simulink model "QET_KV"  (R2015b)
settings: Solver=ode4  SolverMode=SingleTasking  StartTime=0.0  StopTime=inf  FixedStep=Ts  RelTol=1e-3
values from neighbouring files (symbols this model uses):
  F_M_Direction = [1 1 1 -1 -1 -1]    [Config_StepperMotor.m]
  NanoCal7342 = [-0.945276141167 14.673559188843 0.251662999392 -14.892200469971 -0.854624807835 0.034513175488 ... (first row only)    [NanoCalibration.m]
  Resolution = (360/200 * 1/64)    (= 0.028125)    [Config_StepperMotor.m]
undefined symbols (not defined in the file or in its folder): AnalogPos_to_deg, anVE, anVE_GBC_Kbi, anVE_GBC_Kbp, anVE_K_int, anVE_Position_Gain_inv, anVE_Saturation, B, Chirp_Amplitude, Chirp_Freq_Max, Chirp_Freq_Min, Chirp_Period, Chirp_Time_Start, Chirp_Type, delay, Delta, DO_DG409_A0, DO_DG409_A1, Driver_Type, HIL, K, K_gyro, Kd, Kp, lambda, mag, Pos_Final, Pos_Init, Pos_Threshold, PSoC_Freq, qc_get_step_size, Stabilization_Period, Test_type, Times, Torque_Threshold, Ts, Ts_loop, VE_Platform, VE_Type
libraries: quarc_library x22, simulink x13, dspsigops x1
(part 2 of 3)

== system QET_KV/Stability Check and Control ==
  Clock : Clock
  Display : Display
  Display1 : Display
  Initial and Final Condition Control : Subsystem
  Stability Check : Subsystem
  To Workspace2 : ToWorkspace  VariableName=is_stable_vec  SampleTime=-1
      settings: Save2DSignal=2-D array (concatenate along first dimension)
  Switch-State : Outport
  Stable Torque : Outport  Port=2
  tag scope: StabCheck_Pos=global, StabCheck_State=global, is_stable_vec=global
  wires:
  Initial and Final Condition Control/2(Stable Torque) -> Stable Torque/1  "PD"
  Clock/1 -> Display/1, Initial and Final Condition Control/1(Clock), Stability Check/2(Clock)
  Stability Check/1(is_stable) -> [is_stable_vec], To Workspace2/1, Initial and Final Condition Control/2(is_stable), Display1/1
  Initial and Final Condition Control/1(Switch-State) -> [StabCheck_State], Switch-State/1
  Initial and Final Condition Control/4(Pos_Final) -> Stability Check/1(Pos_Final)
  Initial and Final Condition Control/3(Pos_PD) -> [StabCheck_Pos]

== system QET_KV/Step with Rate Limiter ==
  In1 : Inport
  Add1 : Sum  Inputs=+-
  Constant7 : Constant  Value=0
  Manual Switch2 : ManualSwitch
  Multiport Switch2 : MultiPortSwitch  Inputs=2  DataPortForDefault=Additional data port  SampleTime=Ts
  Pulse : Scope
  Rate Limiter : RateLimiter  RisingSlewLimit=100 * pi/180  FallingSlewLimit=-100 * pi/180  SampleTimeMode=inherited
  Scope1 : Scope
  Scope2 : Scope
  Out1 : Outport
  wires:
  In1/1 -> Add1/1, Multiport Switch2/2
  Multiport Switch2/1 -> Scope2/1, Manual Switch2/2, Rate Limiter/1
  Add1/1 -> Pulse/1, Out1/1
  Constant7/1 -> Multiport Switch2/4, Multiport Switch2/3
  [StabCheck_State] -> Scope1/1, Multiport Switch2/1
  Rate Limiter/1 -> Manual Switch2/1
  Manual Switch2/1 -> Add1/2

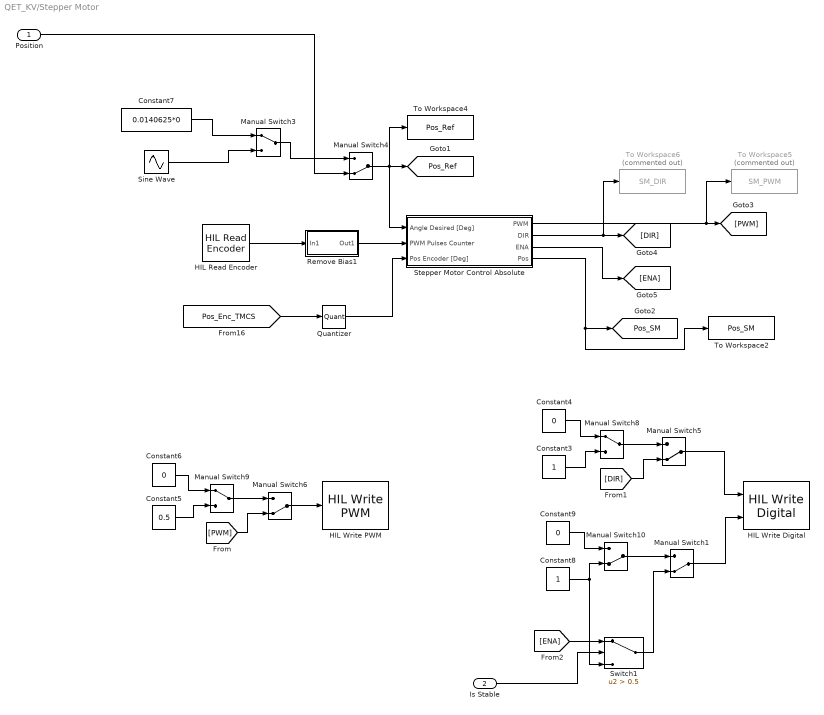
== system QET_KV/Stepper Motor ==
  Position : Inport
  Is Stable : Inport  Port=2
  Constant3 : Constant
  Constant4 : Constant  Value=0
  Constant5 : Constant  Value=0.5
  Constant6 : Constant  Value=0
  Constant7 : Constant  Value=0.0140625*0
  Constant8 : Constant
  Constant9 : Constant  Value=0
  HIL Read Encoder : quarc_library/Data Acquisition/Generic/Immediate I//O/HIL Read Encoder  object_name=HIL-1  channels=[0]  sample_time=qc_get_step_size  active=on  vector_output=off  data_type_mode=Inherit via back propagation  data_type=double
  HIL Write Digital : quarc_library/Data Acquisition/Generic/Immediate I//O/HIL Write Digital  object_name=HIL-1  channels=[0 7]  sample_time=-1  active=off  vector_input=off
  HIL Write PWM : quarc_library/Data Acquisition/Generic/Immediate I//O/HIL Write PWM  object_name=HIL-1  channels=[1]  sample_time=Ts  active=off  vector_input=off
      settings: AttributesFormatString=(%<object_name>)
  Manual Switch{1,4..6,10} (5 alike) : ManualSwitch  CurrentSetting=0
  Manual Switch3 : ManualSwitch
  Manual Switch8 : ManualSwitch
  Manual Switch9 : ManualSwitch
  Quantizer : Quantizer  QuantizationInterval=Resolution  SampleTime=Ts
  Remove Bias1 : Subsystem
  Sine Wave : Sin  Amplitude=0.0140625*5  Frequency=2*pi*1  SampleTime=0
  Stepper Motor Control Absolute : Subsystem
  Switch1 : Switch  Criteria=u2 > Threshold  Threshold=0.5
  To Workspace2 : ToWorkspace  VariableName=Pos_SM  SampleTime=-1
      settings: Save2DSignal=2-D array (concatenate along first dimension)
  To Workspace4 : ToWorkspace  VariableName=Pos_Ref  SampleTime=-1
      settings: Save2DSignal=2-D array (concatenate along first dimension)
  To Workspace5 : ToWorkspace  Commented=on  VariableName=SM_PWM  SampleTime=-1
      settings: Save2DSignal=2-D array (concatenate along first dimension)
  To Workspace6 : ToWorkspace  Commented=on  VariableName=SM_DIR  SampleTime=-1
      settings: Save2DSignal=2-D array (concatenate along first dimension)
  tag scope: Pos_Ref=global, Pos_SM=global
  wires:
  Manual Switch9/1 -> Manual Switch6/1
  Manual Switch3/1 -> Manual Switch4/1
  Manual Switch8/1 -> Manual Switch5/1
  Manual Switch5/1 -> HIL Write Digital/1
  Manual Switch6/1 -> HIL Write PWM/1
  Sine Wave/1 -> Manual Switch3/2
  [PWM] -> Manual Switch6/2
  [DIR] -> Manual Switch5/2
  Manual Switch4/1 -> [Pos_Ref], Stepper Motor Control Absolute/1(Angle Desired [Deg]), To Workspace4/1
  Stepper Motor Control Absolute/1(PWM) -> [PWM], To Workspace5/1
  Stepper Motor Control Absolute/2(DIR) -> [DIR], To Workspace6/1
  HIL Read Encoder/1 -> Remove Bias1/1(In1)
  Stepper Motor Control Absolute/4(Pos) -> To Workspace2/1, [Pos_SM]
  Position/1 -> Manual Switch4/2
  Constant7/1 -> Manual Switch3/1
  Remove Bias1/1(Out1) -> Stepper Motor Control Absolute/2(PWM Pulses Counter)
  [Pos_Enc_TMCS] -> Quantizer/1
  Quantizer/1 -> Stepper Motor Control Absolute/3(Pos Encoder [Deg])
  Constant3/1 -> Manual Switch8/2
  Constant4/1 -> Manual Switch8/1
  Constant6/1 -> Manual Switch9/1
  Constant5/1 -> Manual Switch9/2
  Constant9/1 -> Manual Switch10/1
  Manual Switch10/1 -> Manual Switch1/1
  Manual Switch1/1 -> HIL Write Digital/2
  Stepper Motor Control Absolute/3(ENA) -> [ENA]
  Constant8/1 -> Switch1/3, Manual Switch10/2
  [ENA] -> Switch1/1
  Is Stable/1 -> Switch1/2
  Switch1/1 -> Manual Switch1/2

== system QET_KV/Time Enable1 ==
  In1 : Inport
  Product2 : Product  Inputs=3
  Step4 : Step  Time=Chirp_Time_Start-0.007  SampleTime=Ts
  Step5 : Step  Time=Chirp_Period+1.5  Before=1  After=0  SampleTime=Ts
  Out1 : Outport
  wires:
  Step5/1 -> Product2/3
  Product2/1 -> Out1/1
  In1/1 -> Product2/1
  Step4/1 -> Product2/2

== system QET_KV/Torques ==
  Display : Display
  Gain : Gain  Gain=-1
  Mux1 : Mux  Inputs=2
  Mux2 : Mux  Inputs=2
  Mux6 : Mux
  Torque F/T Sensor : Scope
  Torques : Scope
  Voltage Applied : Scope
  wires:
  Mux6/1 -> Display/1, Torques/1
  [Torque_Haptic] -> Mux6/1  "VE"
  [Torque_Current_QET2] -> Mux6/2  "Current QET2"
  [Torque_Current_AMC] -> Mux6/3  "Current AMC"
  [Torque_Current_CD1] -> Mux6/4  "Current CD1"
  Mux1/1 -> Torque F/T Sensor/1
  [Torque_Current_CD1] -> Mux1/2
  [Torque_Nano25] -> Gain/1
  Gain/1 -> Mux1/1
  [anVE_Output_Voltage] -> Mux2/1
  [DC_Motor_Analog] -> Mux2/2
  Mux2/1 -> Voltage Applied/1

== system QET_KV/Virtual Environment ==
  Position : Inport
  Constant10 : Constant
  Constant5 : Constant  Value=delay
  Constant9 : Constant  Value=VE_Type
  Deg to Rad : Gain  Gain=pi/180
  Force VE Delay : Scope
  Manual Switch2 : ManualSwitch
  Manual Switch4 : ManualSwitch
  Multiport Switch2 : MultiPortSwitch  DataPortForDefault=Additional data port  SampleTime=Ts
  Mux7 : Mux  Inputs=2
  To Workspace1 : ToWorkspace  VariableName=Torque_VE_Both  SampleTime=-1
      settings: Save2DSignal=2-D array (concatenate along first dimension)
  To Workspace3 : ToWorkspace  VariableName=Torque_VE  SaveFormat=Structure With Time  SampleTime=-1
  VE_KV_BD : Subsystem
  VE_KV_GM2 : Subsystem
  VE_PV : Subsystem
  Variable Integer Delay : Delay  DelayLengthSource=Input port  DelayLengthUpperLimit=20
      settings: InputPortMap=u0,p1
  Torque : Outport
  tag scope: Torque_VE=global
  wires:
  VE_KV_BD/1(Torque) -> Multiport Switch2/2
  VE_KV_GM2/1(Torque) -> Multiport Switch2/5, Multiport Switch2/3
  Position/1 -> VE_PV/1(Position), VE_KV_GM2/1(Position), VE_KV_BD/1(Position)
  Multiport Switch2/1 -> Variable Integer Delay/1, Mux7/1, Manual Switch2/2
  Variable Integer Delay/1 -> Mux7/2, Manual Switch2/1
  Manual Switch2/1 -> Torque/1, [Torque_VE], To Workspace3/1
  Constant5/1 -> Variable Integer Delay/2
  Mux7/1 -> To Workspace1/1, Force VE Delay/1
  VE_PV/1(Torque) -> Multiport Switch2/4
  Constant9/1 -> Manual Switch4/1
  Constant10/1 -> Manual Switch4/2
  Manual Switch4/1 -> Multiport Switch2/1
  [Velocity_Gyro] -> Deg to Rad/1
  Deg to Rad/1 -> VE_PV/2(Velocity)

== system QET_KV/Analog Inputs (Analog VE)/Remove Bias w LPF ==
  In1 : Inport
  Step : Step  Time=.15  Before=1  After=0  SampleTime=qc_get_step_size
  Sum1 : Sum  Inputs=|+-
  Switch : Switch  Criteria=u2 > Threshold  Threshold=0.5  SampleTime=qc_get_step_size
  Transfer Fcn : TransferFcn  Denominator=[1/(2*pi*50) 1]
  Unit Delay : UnitDelay  SampleTime=-1
  Out1 : Outport
  wires:
  In1/1 -> Switch/1, Sum1/1
  Step/1 -> Switch/2
  Unit Delay/1 -> Switch/3
  Sum1/1 -> Out1/1
  Switch/1 -> Transfer Fcn/1, Sum1/2
  Transfer Fcn/1 -> Unit Delay/1

== system QET_KV/Analog Inputs (Analog VE)/Remove Bias2 ==
  In1 : Inport
  Step : Step  Time=.15  Before=1  After=0  SampleTime=qc_get_step_size
  Sum1 : Sum  Inputs=|+-
  Switch : Switch  Criteria=u2 > Threshold  Threshold=0.5  SampleTime=qc_get_step_size
  Unit Delay : UnitDelay  SampleTime=-1
  Out1 : Outport
  wires:
  In1/1 -> Switch/1, Sum1/1
  Switch/1 -> Unit Delay/1, Sum1/2
  Step/1 -> Switch/2
  Unit Delay/1 -> Switch/3
  Sum1/1 -> Out1/1

== system QET_KV/Analog Inputs (Analog VE)/Remove Bias6 ==
  In1 : Inport
  Step : Step  Time=.2  Before=1  After=0  SampleTime=Ts
  Sum1 : Sum  Inputs=|+-  SampleTime=Ts
  Switch : Switch  Criteria=u2 > Threshold  Threshold=0.5  SampleTime=Ts
  Unit Delay : UnitDelay  SampleTime=Ts
  Out1 : Outport
  wires:
  In1/1 -> Switch/1, Sum1/1
  Switch/1 -> Unit Delay/1, Sum1/2
  Step/1 -> Switch/2
  Unit Delay/1 -> Switch/3
  Sum1/1 -> Out1/1

== system QET_KV/Analog Inputs (Digital VE)/Remove Bias w LPF ==
  In1 : Inport
  Step : Step  Time=.15  Before=1  After=0  SampleTime=qc_get_step_size
  Sum1 : Sum  Inputs=|+-
  Switch : Switch  Criteria=u2 > Threshold  Threshold=0.5  SampleTime=qc_get_step_size
  Transfer Fcn : TransferFcn  Denominator=[1/(2*pi*50) 1]
  Unit Delay : UnitDelay  SampleTime=-1
  Out1 : Outport
  wires:
  In1/1 -> Switch/1, Sum1/1
  Step/1 -> Switch/2
  Unit Delay/1 -> Switch/3
  Sum1/1 -> Out1/1
  Switch/1 -> Transfer Fcn/1, Sum1/2
  Transfer Fcn/1 -> Unit Delay/1

== system QET_KV/Analog Inputs (Digital VE)/Remove Bias2 ==
  In1 : Inport
  Step : Step  Time=.15  Before=1  After=0  SampleTime=qc_get_step_size
  Sum1 : Sum  Inputs=|+-
  Switch : Switch  Criteria=u2 > Threshold  Threshold=0.5  SampleTime=qc_get_step_size
  Unit Delay : UnitDelay  SampleTime=-1
  Out1 : Outport
  wires:
  In1/1 -> Switch/1, Sum1/1
  Switch/1 -> Unit Delay/1, Sum1/2
  Step/1 -> Switch/2
  Unit Delay/1 -> Switch/3
  Sum1/1 -> Out1/1

== system QET_KV/Analog Inputs (Digital VE)/Remove Bias5 ==
  In1 : Inport
  Step : Step  Time=.15  Before=1  After=0  SampleTime=qc_get_step_size
  Sum1 : Sum  Inputs=|+-
  Switch : Switch  Criteria=u2 > Threshold  Threshold=0.5  SampleTime=qc_get_step_size
  Unit Delay : UnitDelay  SampleTime=-1
  Out1 : Outport
  wires:
  In1/1 -> Switch/1, Sum1/1
  Switch/1 -> Unit Delay/1, Sum1/2
  Step/1 -> Switch/2
  Unit Delay/1 -> Switch/3
  Sum1/1 -> Out1/1

== system QET_KV/Analog Inputs (Digital VE)/Remove Bias6 ==
  In1 : Inport
  Step : Step  Time=.15  Before=1  After=0  SampleTime=qc_get_step_size
  Sum1 : Sum  Inputs=|+-
  Switch : Switch  Criteria=u2 > Threshold  Threshold=0.5  SampleTime=qc_get_step_size
  Unit Delay : UnitDelay  SampleTime=-1
  Out1 : Outport
  wires:
  In1/1 -> Switch/1, Sum1/1
  Switch/1 -> Unit Delay/1, Sum1/2
  Step/1 -> Switch/2
  Unit Delay/1 -> Switch/3
  Sum1/1 -> Out1/1

== system QET_KV/Analog VE/Digital Outputs ==
  Clock Pulses : Subsystem  Commented=on
  Constant1 : Constant  Value=0.1
  Constant11 : Constant  Commented=on  Value=0
  Constant12 : Constant  Value=Chirp_Time_Start
  Constant13 : Constant  Value=Times(4)
  Constant2 : Constant  Value=0.1
  Constant4 : Constant
  Constant5 : Constant  Value=0
  Constant8 : Constant  Commented=on  Value=0.9
  Constant9 : Constant  Commented=on  Value=Chirp_Time_Start
  Goto3 : Goto  Commented=on  GotoTag=DO_10  TagVisibility=global
  Goto4 : Goto  Commented=on  GotoTag=DO_11  TagVisibility=global
  Position Switch2 : ManualSwitch  CurrentSetting=0
  Position Switch5 : ManualSwitch  Commented=on
  Position Switch6 : ManualSwitch  Commented=on
  Pulse : Subsystem
  Time Enable2 : Subsystem  Commented=on
  Unit Pulse : Subsystem  Commented=on
  Unit Pulse1 : Subsystem
  tag scope: DO_Reset_ENC=global, DO_Trigger=global
  wires:
  Unit Pulse/1(Out1) -> Goto3/1
  Constant8/1 -> Clock Pulses/1(Time [s]), Unit Pulse/1(Time [s])
  Constant9/1 -> Clock Pulses/2(Width [s]), Unit Pulse/2(Width [s])
  Position Switch6/1 -> Goto4/1
  Clock Pulses/1(Out1) -> Position Switch6/1
  Constant11/1 -> Position Switch6/2
  Time Enable2/1(Out1) -> Position Switch5/1
  Constant12/1 -> Unit Pulse1/1(Time [s])
  Unit Pulse1/1(Out1) -> [DO_Trigger]
  Constant1/1 -> Unit Pulse1/2(Width [s])
  Constant13/1 -> Pulse/3(Width [s])
  Constant2/1 -> Pulse/2(Time [s])
  Pulse/1(Out1) -> [DO_Reset_ENC]
  Constant4/1 -> Position Switch2/2
  Constant5/1 -> Position Switch2/1
  Position Switch2/1 -> Pulse/1(Amplitude)  "IN2"

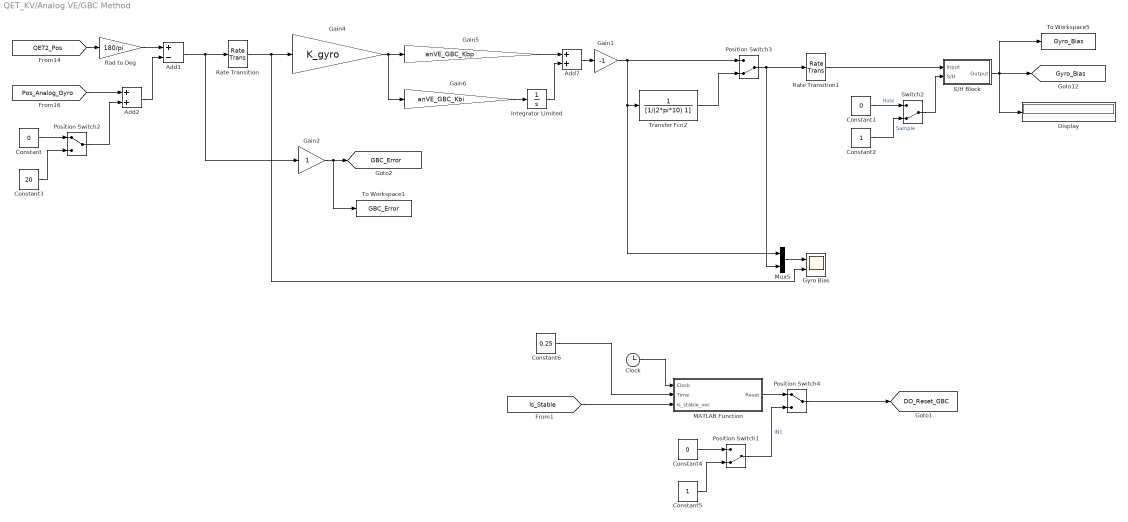
== system QET_KV/Analog VE/GBC Method ==
  Add1 : Sum  Inputs=+-
  Add2 : Sum
  Add7 : Sum
  Clock : Clock
  Constant : Constant  Value=0
  Constant1 : Constant  Value=0
  Constant2 : Constant
  Constant3 : Constant  Value=20
  Constant4 : Constant  Value=0
  Constant5 : Constant
  Constant6 : Constant  Value=0.25
  Display : Display
  Gain1 : Gain  Gain=-1
  Gain2 : Gain
  Gain4 : Gain  Gain=K_gyro
  Gain5 : Gain  Gain=anVE_GBC_Kbp
  Gain6 : Gain  Gain=anVE_GBC_Kbi
  Gyro Bias : Scope  NumInputPorts=2
  Integrator Limited : Integrator  LimitOutput=on  UpperSaturationLimit=0.05  LowerSaturationLimit=-0.05
  MATLAB Function : MATLAB Function  TreatAsAtomicUnit=on
  Mux5 : Mux  Inputs=2
  Position Switch1 : ManualSwitch  CurrentSetting=0
  Position Switch2 : ManualSwitch
  Position Switch3 : ManualSwitch  CurrentSetting=0
  Position Switch4 : ManualSwitch
  "Rad to Deg " : Gain  Gain=180/pi
  Rate Transition : RateTransition  Integrity=off  Deterministic=off  OutPortSampleTime=Ts_loop
  Rate Transition1 : RateTransition  Integrity=off  Deterministic=off  OutPortSampleTime=Ts
  S/H Block : Subsystem
  Switch2 : ManualSwitch  CurrentSetting=0
  To Workspace1 : ToWorkspace  VariableName=GBC_Error  SampleTime=-1
      settings: Save2DSignal=2-D array (concatenate along first dimension)
  To Workspace5 : ToWorkspace  VariableName=Gyro_Bias  SampleTime=-1
      settings: Save2DSignal=2-D array (concatenate along first dimension)
  Transfer Fcn2 : TransferFcn  Denominator=[1/(2*pi*10) 1]
  tag scope: DO_Reset_GBC=global, GBC_Error=global, Gyro_Bias=global
  wires:
  Gain6/1 -> Integrator Limited/1
  Add7/1 -> Gain1/1
  Gain4/1 -> Gain6/1, Gain5/1
  Gain5/1 -> Add7/1
  Integrator Limited/1 -> Add7/2
  [QET2_Pos] -> "Rad to Deg "/1
  Gain1/1 -> Transfer Fcn2/1, Mux5/1, Position Switch3/1
  "Rad to Deg "/1 -> Add1/1
  Constant1/1 -> Switch2/1  "Hold"
  Constant2/1 -> Switch2/2  "Sample"
  Switch2/1 -> S/H Block/2(S/H)
  S/H Block/1(Output) -> Display/1, To Workspace5/1, [Gyro_Bias]
  Position Switch3/1 -> Rate Transition1/1, Mux5/2
  Mux5/1 -> Gyro Bias/1
  Add1/1 -> Gain2/1, Rate Transition/1
  Constant/1 -> Position Switch2/1
  Constant3/1 -> Position Switch2/2
  [Pos_Analog_Gyro] -> Add2/1
  Add2/1 -> Add1/2
  Position Switch2/1 -> Add2/2
  Constant5/1 -> Position Switch1/2
  Constant4/1 -> Position Switch1/1
  Position Switch4/1 -> [DO_Reset_GBC]
  MATLAB Function/1(Reset) -> Position Switch4/1
  Position Switch1/1 -> Position Switch4/2  "IN1"
  Clock/1 -> MATLAB Function/1(Clock)
  Constant6/1 -> MATLAB Function/2(Time)
  [Is_Stable] -> MATLAB Function/3(is_stable_vec)
  Transfer Fcn2/1 -> Position Switch3/2
  Rate Transition/1 -> Gain4/1, Gyro Bias/2
  Rate Transition1/1 -> S/H Block/1(Input)
  Gain2/1 -> To Workspace1/1, [GBC_Error]

== system QET_KV/Analog VE/GBC Method -WHC ==
  Add1 : Sum  Inputs=+-
  Add7 : Sum
  Constant1 : Constant  Value=0
  Constant2 : Constant
  Display : Display
  Gain1 : Gain  Gain=-1
  Gain4 : Gain  Gain=K_gyro/anVE_K_int
  Gain5 : Gain  Gain=anVE.Kbias_p
  Gain6 : Gain  Gain=anVE.Kbias_i
  Gyro Bias : Scope  NumInputPorts=2
  Integrator Limited : Integrator  LimitOutput=on  UpperSaturationLimit=0.5  LowerSaturationLimit=-0.5
  Mux5 : Mux  Inputs=2
  Position Switch3 : ManualSwitch  CurrentSetting=0
  "Rad to Deg " : Gain  Gain=180/pi
  S/H Block : Subsystem
  Switch2 : ManualSwitch  CurrentSetting=0
  To Workspace5 : ToWorkspace  VariableName=Gyro_Bias  SampleTime=-1
      settings: Save2DSignal=2-D array (concatenate along first dimension)
  Transfer Fcn2 : TransferFcn  Denominator=[1/(2*pi*10) 1]
  tag scope: Gyro_Bias=global
  wires:
  Gain6/1 -> Integrator Limited/1
  Add7/1 -> Gain1/1
  Gain4/1 -> Gain6/1, Gain5/1
  Gain5/1 -> Add7/1
  Integrator Limited/1 -> Add7/2
  [Pos_Analog_Gyro] -> Add1/2
  [QET2_Pos] -> "Rad to Deg "/1
  Transfer Fcn2/1 -> Position Switch3/2
  Gain1/1 -> Transfer Fcn2/1, Mux5/1, Position Switch3/1
  "Rad to Deg "/1 -> Add1/1
  Constant1/1 -> Switch2/1  "Hold"
  Constant2/1 -> Switch2/2  "Sample"
  Switch2/1 -> S/H Block/2(S/H)
  S/H Block/1(Output) -> Display/1, To Workspace5/1, [Gyro_Bias]
  Position Switch3/1 -> S/H Block/1(Input), Mux5/2
  Mux5/1 -> Gyro Bias/1
  Add1/1 -> Gyro Bias/2, Gain4/1

== system QET_KV/Analog VE/Remove Bias1 ==
  In1 : Inport
  Step : Step  Time=.2  Before=1  After=0  SampleTime=Ts
  Sum1 : Sum  Inputs=|+-  SampleTime=Ts
  Switch : Switch  Criteria=u2 > Threshold  Threshold=0.5  SampleTime=Ts
  Unit Delay : UnitDelay  SampleTime=Ts
  Out1 : Outport
  wires:
  In1/1 -> Switch/1, Sum1/1
  Switch/1 -> Unit Delay/1, Sum1/2
  Step/1 -> Switch/2
  Unit Delay/1 -> Switch/3
  Sum1/1 -> Out1/1

== system QET_KV/Chirp and White Noise/Chirp 1 ==
  Clock : Clock
  Constant1 : Constant  Value=Chirp_Freq_Min
  Constant2 : Constant  Value=Chirp_Freq_Max
  Constant3 : Constant  Value=Chirp_Period
  Constant4 : Constant  Value=Chirp_Time_Start
  Constant5 : Constant  Value=Chirp_Type
  Constant6 : Constant
  MATLAB Function : MATLAB Function  TreatAsAtomicUnit=on
  Sine : Outport
  Freq : Outport  Port=2
  wires:
  Constant2/1 -> MATLAB Function/7(fmax)
  Clock/1 -> MATLAB Function/2(clock)
  Constant1/1 -> MATLAB Function/6(fmin)
  MATLAB Function/1(y) -> Sine/1
  Constant3/1 -> MATLAB Function/3(chirp_period)
  MATLAB Function/2(f) -> Freq/1
  Constant4/1 -> MATLAB Function/4(chirp_start)
  Constant5/1 -> MATLAB Function/1(type)
  Constant6/1 -> MATLAB Function/5(chirp_amp)

== system QET_KV/Chirp and White Noise/PI Controller ==
  Ref 1 : Inport
  Ref 2 : Inport  Port=2
  Input : Inport  Port=3
  Add1 : Sum  Inputs=++-
  Add2 : Sum
  Constant4 : Constant  Value=49.99  VectorParams1D=off
  Display1 : Display
  Gain1 : Gain  Gain=0
  Gain4 : Gain  Gain=1000
  Gain5 : Gain  Gain=2.5
  Integrator : Integrator  ExternalReset=level
  Mux1 : Mux  Inputs=2
  PI Output : Scope  NumInputPorts=2
  Product4 : Product
  Relational Operator1 : RelationalOperator  OutDataTypeStr=boolean
  Step1 : Step  Time=Chirp_Time_Start
  Transfer Fcn : TransferFcn  Denominator=[1/(2*pi*1) 1]
  Transfer Fcn3 : TransferFcn  Denominator=[1/(2*pi*.1) 1]
  Gain out : Outport
  wires:
  Input/1 -> Add1/3
  Ref 2/1 -> Gain1/1
  Step1/1 -> Transfer Fcn/1
  Ref 1/1 -> Add1/1
  Integrator/1 -> Gain5/1
  Gain5/1 -> Display1/1, Mux1/2, Add2/2  "Integral"
  Gain4/1 -> Mux1/1, Add2/1  "Proportional"
  Add2/1 -> Transfer Fcn3/1
  Transfer Fcn3/1 -> PI Output/2, Gain out/1, Relational Operator1/1  "Output Filtered"
  Add1/1 -> Product4/2
  Product4/1 -> Gain4/1, Integrator/1
  Transfer Fcn/1 -> Product4/1
  Constant4/1 -> Relational Operator1/2
  Relational Operator1/1 -> Integrator/2
  Gain1/1 -> Add1/2
  Mux1/1 -> PI Output/1

== system QET_KV/Enc Position Inputs/Remove Bias1 ==
  In1 : Inport
  Step : Step  Time=.2  Before=1  After=0  SampleTime=Ts
  Sum1 : Sum  Inputs=|+-  SampleTime=Ts
  Switch : Switch  Criteria=u2 > Threshold  Threshold=0.5  SampleTime=Ts
  Unit Delay : UnitDelay  SampleTime=Ts
  Out1 : Outport
  wires:
  In1/1 -> Switch/1, Sum1/1
  Switch/1 -> Unit Delay/1, Sum1/2
  Step/1 -> Switch/2
  Unit Delay/1 -> Switch/3
  Sum1/1 -> Out1/1

== system QET_KV/Enc Position Inputs/Remove Bias3 ==
  In1 : Inport
  Step : Step  Time=0.2  Before=1  After=0  SampleTime=Ts
  Sum1 : Sum  Inputs=|+-
  Switch : Switch  Criteria=u2 > Threshold  Threshold=0.5
  Unit Delay : UnitDelay  SampleTime=-1
  Out1 : Outport
  wires:
  In1/1 -> Switch/1, Sum1/1
  Switch/1 -> Unit Delay/1, Sum1/2
  Step/1 -> Switch/2
  Unit Delay/1 -> Switch/3
  Sum1/1 -> Out1/1

== system QET_KV/Enc Position Inputs/Remove Bias4 ==
  In1 : Inport
  Step : Step  Time=0.2  Before=1  After=0  SampleTime=Ts
  Sum1 : Sum  Inputs=|+-
  Switch : Switch  Criteria=u2 > Threshold  Threshold=0.5
  Unit Delay : UnitDelay  SampleTime=-1
  Out1 : Outport
  wires:
  In1/1 -> Switch/1, Sum1/1
  Switch/1 -> Unit Delay/1, Sum1/2
  Step/1 -> Switch/2
  Unit Delay/1 -> Switch/3
  Sum1/1 -> Out1/1

== system QET_KV/General Output/Bias ==
  In1 : Inport
  Constant : Constant  Value=0
  Sum1 : Sum  Inputs=|++
  Out1 : Outport
  wires:
  In1/1 -> Sum1/1
  Constant/1 -> Sum1/2
  Sum1/1 -> Out1/1

== system QET_KV/General Output/Bias1 ==
  In1 : Inport
  Constant : Constant  Value=-0.0012*8
  Sum1 : Sum  Inputs=|++
  Out1 : Outport
  wires:
  In1/1 -> Sum1/1
  Constant/1 -> Sum1/2
  Sum1/1 -> Out1/1

== system QET_KV/General Output/Bias2 ==
  In1 : Inport
  Constant : Constant  Value=0
  Sum1 : Sum  Inputs=|++
  Out1 : Outport
  wires:
  In1/1 -> Sum1/1
  Constant/1 -> Sum1/2
  Sum1/1 -> Out1/1

== system QET_KV/General Output/Reset ERG Square Signal ==
  Gain : Gain
  Logical Operator : Logic  Operator=NOT  AllPortsSameDT=off  OutDataTypeStr=boolean
  Memory : Memory
  Rate Transition2 : RateTransition  Integrity=off  Deterministic=off  OutPortSampleTime=Ts_loop
  Rate Transition3 : RateTransition  Integrity=off  Deterministic=off  OutPortSampleTime=Ts
  Out1 : Outport
  wires:
  Memory/1 -> Logical Operator/1
  Logical Operator/1 -> Rate Transition2/1
  Rate Transition2/1 -> Gain/1
  Gain/1 -> Rate Transition3/1
  Rate Transition3/1 -> Memory/1, Out1/1

== system QET_KV/General Output/Time Enable2 ==
  In1 : Inport
  Product2 : Product  Inputs=3
  Step4 : Step  Time=0.1  SampleTime=Ts
  Step5 : Step  Time=Chirp_Period+1.5  Before=1  After=0  SampleTime=Ts
  Out1 : Outport
  wires:
  Step5/1 -> Product2/3
  Product2/1 -> Out1/1
  In1/1 -> Product2/1
  Step4/1 -> Product2/2

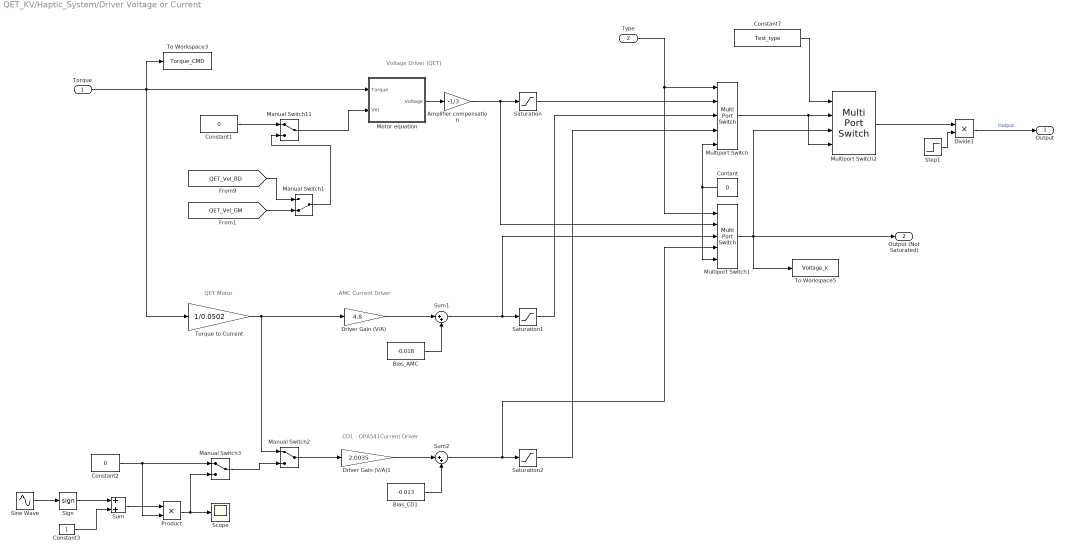
== system QET_KV/Haptic_System/Driver Voltage or Current ==
  note: Voltage Driver (QET)
  note: AMC Current Driver
  note: QET Motor
  note: CD1 - OPA541Current Driver
  Torque : Inport
  Type : Inport  Port=2
  Amplifier compensation : Gain  Gain=-1/3
  Bias_AMC : Constant  Value=-0.018
  Bias_CD1 : Constant  Value=-0.013
  Constant1 : Constant  Value=0
  Constant2 : Constant  Value=0
  Constant3 : Constant
  Constant7 : Constant  Value=Test_type
  Contant : Constant  Value=0  SampleTime=Ts
  Divide1 : Product  Inputs=**  SampleTime=Ts
  Driver Gain (V/A) : Gain  Gain=4.8
  Driver Gain (V/A)1 : Gain  Gain=2.0035
  Manual Switch1 : ManualSwitch  CurrentSetting=0
  Manual Switch11 : ManualSwitch
  Manual Switch2 : ManualSwitch
  Manual Switch3 : ManualSwitch
  Motor equation : Subsystem
  Multiport Switch : MultiPortSwitch  DataPortForDefault=Additional data port
  Multiport Switch1 : MultiPortSwitch  DataPortForDefault=Additional data port
  Multiport Switch2 : MultiPortSwitch  DataPortOrder=Specify indices  Inputs=1  DataPortIndices={[1,2,3,4],5}  DataPortForDefault=Additional data port
  Product : Product
  Saturation : Saturate  UpperLimit=4.5  LowerLimit=-4.5
  Saturation1 : Saturate  UpperLimit=5  LowerLimit=-5
  Saturation2 : Saturate  UpperLimit=2  LowerLimit=-2
  Scope : Scope
  Sign : Signum
  Sine Wave : Sin  Frequency=2*pi*1  SampleTime=0
  Step1 : Step  Time=0.1  SampleTime=Ts
  Sum : Sum
  Sum1 : Sum  Inputs=|++
  Sum2 : Sum  Inputs=|++
  To Workspace3 : ToWorkspace  VariableName=Torque_CMD  SampleTime=-1
      settings: Save2DSignal=2-D array (concatenate along first dimension)
  To Workspace5 : ToWorkspace  VariableName=Voltage_k  SampleTime=-1
      settings: Save2DSignal=2-D array (concatenate along first dimension)
  Torque to Current : Gain  Gain=1/0.0502  SampleTime=Ts
  Output : Outport
  Output (Not Saturated) : Outport  Port=2
  wires:
  Motor equation/1(Voltage) -> Amplifier compensation/1
  Amplifier compensation/1 -> Multiport Switch1/2, Saturation/1
  Divide1/1 -> Output/1  "Output"
  Step1/1 -> Divide1/2
  Type/1 -> Multiport Switch1/1, Multiport Switch/1
  Saturation/1 -> Multiport Switch/2
  Multiport Switch1/1 -> Multiport Switch2/3, Output (Not Saturated)/1, To Workspace5/1
  Torque to Current/1 -> Driver Gain (V/A)/1, Manual Switch2/1
  Contant/1 -> Multiport Switch/5, Multiport Switch1/5
  Saturation1/1 -> Multiport Switch/3
  Torque/1 -> Motor equation/1(Torque), To Workspace3/1, Torque to Current/1
  Saturation2/1 -> Multiport Switch/4
  Sum1/1 -> Saturation1/1, Multiport Switch1/3
  Sum2/1 -> Saturation2/1, Multiport Switch1/4
  Driver Gain (V/A)/1 -> Sum1/1
  Bias_AMC/1 -> Sum1/2
  Driver Gain (V/A)1/1 -> Sum2/1
  Bias_CD1/1 -> Sum2/2
  Constant1/1 -> Manual Switch11/1
  Manual Switch11/1 -> Motor equation/2(Vel)
  [QET_Vel_BD] -> Manual Switch1/1
  [QET_Vel_GM] -> Manual Switch1/2
  Manual Switch1/1 -> Manual Switch11/2
  Manual Switch2/1 -> Driver Gain (V/A)1/1
  Constant2/1 -> Product/2, Manual Switch3/1
  Manual Switch3/1 -> Manual Switch2/2
  Sine Wave/1 -> Sign/1
  Product/1 -> Manual Switch3/2, Scope/1
  Sign/1 -> Sum/1
  Sum/1 -> Product/1
  Constant3/1 -> Sum/2
  Multiport Switch2/1 -> Divide1/1
  Constant7/1 -> Multiport Switch2/1
  Multiport Switch/1 -> Multiport Switch2/4, Multiport Switch2/2

== system QET_KV/PSoC Comm/Init Delay ==
  In1 : Inport
  Constant : Constant  Value=1e-7
  Step1 : Step  Time=0.01  SampleTime=Ts
  Switch : Switch  Criteria=u2 > Threshold  Threshold=0.5  SampleTime=Ts
  Out1 : Outport
  wires:
  Switch/1 -> Out1/1
  Step1/1 -> Switch/2
  Constant/1 -> Switch/3
  In1/1 -> Switch/1

== system QET_KV/PSoC Comm/Init Delay1 ==
  In1 : Inport
  Divide1 : Product  Inputs=**  SampleTime=Ts
  Step1 : Step  Time=0.22  SampleTime=Ts
  Out1 : Outport
  wires:
  Step1/1 -> Divide1/2
  In1/1 -> Divide1/1
  Divide1/1 -> Out1/1

== system QET_KV/PSoC Comm/Init Delay2 ==
  In1 : Inport
  Divide1 : Product  Inputs=**  SampleTime=Ts
  Step1 : Step  Time=0.35  SampleTime=Ts
  Out1 : Outport
  wires:
  Step1/1 -> Divide1/2
  In1/1 -> Divide1/1
  Divide1/1 -> Out1/1

== system QET_KV/PSoC Comm/Init Delay3 ==
  In1 : Inport
  Constant : Constant  Value=1e-7
  Step1 : Step  Time=0.11  SampleTime=Ts
  Switch : Switch  Criteria=u2 > Threshold  Threshold=0.5  SampleTime=Ts
  Out1 : Outport
  wires:
  Switch/1 -> Out1/1
  Step1/1 -> Switch/2
  Constant/1 -> Switch/3
  In1/1 -> Switch/1

== system QET_KV/Panto A - Force_LP_v2/Axis Selector1 ==
  Forces [6x1] : Inport
  Demux : Demux  Outputs=6
  Mux : Mux  Inputs=3
  Terminator : Terminator
  Terminator1 : Terminator
  Terminator2 : Terminator
  Forces [3x1] : Outport
  wires:
  Demux/6 -> Mux/3
  Forces [6x1]/1 -> Demux/1
  Mux/1 -> Forces [3x1]/1
  Demux/1 -> Terminator/1
  Demux/2 -> Terminator1/1
  Demux/3 -> Terminator2/1
  Demux/4 -> Mux/1
  Demux/5 -> Mux/2

== system QET_KV/Panto A - Force_LP_v2/Axis Selector2 ==
  Forces [6x1] : Inport
  Demux : Demux  Outputs=6
  Mux : Mux  Inputs=3
  Terminator : Terminator
  Terminator1 : Terminator
  Terminator2 : Terminator
  Forces [3x1] : Outport
  wires:
  Demux/1 -> Mux/1
  Demux/2 -> Mux/2
  Demux/6 -> Mux/3
  Forces [6x1]/1 -> Demux/1
  Mux/1 -> Forces [3x1]/1
  Demux/3 -> Terminator/1
  Demux/4 -> Terminator1/1
  Demux/5 -> Terminator2/1

== system QET_KV/Panto A - Force_LP_v2/Discrete Filters ==
  Input [6x1] : Inport
  Axis Direciton : Gain  Gain=F_M_Direction(1)  SaturateOnIntegerOverflow=on  OutDataTypeStr=Inherit: Same as input  ParamDataTypeStr=Inherit: Same as input
  Axis Direciton1 : Gain  Gain=F_M_Direction(2)  SaturateOnIntegerOverflow=on  OutDataTypeStr=Inherit: Same as input  ParamDataTypeStr=Inherit: Same as input
  Axis Direciton2 : Gain  Gain=F_M_Direction(3)  SaturateOnIntegerOverflow=on  OutDataTypeStr=Inherit: Same as input  ParamDataTypeStr=Inherit: Same as input
  Axis Direciton3 : Gain  Gain=F_M_Direction(4)  SaturateOnIntegerOverflow=on  OutDataTypeStr=Inherit: Same as input  ParamDataTypeStr=Inherit: Same as input
  Axis Direciton4 : Gain  Gain=F_M_Direction(5)  SaturateOnIntegerOverflow=on  OutDataTypeStr=Inherit: Same as input  ParamDataTypeStr=Inherit: Same as input
  Axis Direciton5 : Gain  Gain=F_M_Direction(6)  SaturateOnIntegerOverflow=on  OutDataTypeStr=Inherit: Same as input  ParamDataTypeStr=Inherit: Same as input
  Demux : Demux  Outputs=6
  Discrete Transfer Fcn : DiscreteTransferFcn  Commented=through  Numerator=[0.01053 0.0421 0.06315 0.0421 0.01053]  Denominator=[1 -1.438 0.775 -0.1857 0.01668]
  Discrete Transfer Fcn1 : DiscreteTransferFcn  Commented=through  Numerator=[0.01053 0.0421 0.06315 0.0421 0.01053]  Denominator=[1 -1.438 0.775 -0.1857 0.01668]  SampleTime=Ts
  Discrete Transfer Fcn5 : DiscreteTransferFcn  Commented=through  Numerator=[0.01053 0.0421 0.06315 0.0421 0.01053]  Denominator=[1 -1.438 0.775 -0.1857 0.01668]
  Mux1 : Mux  Inputs=6
  Output [6x1] : Outport
  wires:
  Axis Direciton5/1 -> Mux1/6
  Axis Direciton4/1 -> Mux1/5
  Axis Direciton3/1 -> Mux1/4
  Axis Direciton2/1 -> Mux1/3
  Axis Direciton1/1 -> Mux1/2
  Axis Direciton/1 -> Mux1/1
  Demux/1 -> Discrete Transfer Fcn/1
  Discrete Transfer Fcn/1 -> Axis Direciton/1
  Demux/2 -> Discrete Transfer Fcn1/1
  Discrete Transfer Fcn1/1 -> Axis Direciton1/1
  Demux/3 -> Axis Direciton2/1
  Demux/4 -> Axis Direciton3/1
  Demux/5 -> Axis Direciton4/1
  Demux/6 -> Discrete Transfer Fcn5/1
  Input [6x1]/1 -> Demux/1
  Mux1/1 -> Output [6x1]/1
  Discrete Transfer Fcn5/1 -> Axis Direciton5/1

== system QET_KV/Position and Velocities/GM ==
  Pos : Inport
  Add1 : Sum  Inputs=+-  SampleTime=Ts_loop
  Difference : simulink/Discrete/Difference  ICPrevInput=0.0  InputProcessing=Inherited  OutMin=[]  OutMax=[]  OutDataType=fixdt(1, 16)  OutScaling=2^-10  DoSatur=off
  Gain3 : Gain  Gain=1/Delta  SampleTime=Ts_loop
  Gain4 : Gain  Gain=1/mag  SampleTime=Ts_loop
  Gain5 : Gain  Gain=lambda  SampleTime=Ts_loop
  Unit Delay : UnitDelay  SampleTime=Ts_loop
  Vel : Outport
  wires:
  Unit Delay/1 -> Gain5/1
  Difference/1 -> Gain3/1
  Gain5/1 -> Add1/2
  Gain3/1 -> Add1/1
  Gain4/1 -> Vel/1  "GM_2"
  Pos/1 -> Difference/1
  Add1/1 -> Gain4/1, Unit Delay/1

== system QET_KV/Position and Velocities/GM1 ==
  Pos : Inport
  Add1 : Sum  Inputs=+-  SampleTime=Ts_loop
  Difference : simulink/Discrete/Difference  ICPrevInput=0.0  InputProcessing=Inherited  OutMin=[]  OutMax=[]  OutDataType=fixdt(1, 16)  OutScaling=2^-10  DoSatur=off
  Gain3 : Gain  Gain=1/Delta  SampleTime=Ts_loop
  Gain4 : Gain  Gain=1/mag  SampleTime=Ts_loop
  Gain5 : Gain  Gain=lambda  SampleTime=Ts_loop
  Unit Delay : UnitDelay  SampleTime=Ts_loop
  Vel : Outport
  wires:
  Unit Delay/1 -> Gain5/1
  Difference/1 -> Gain3/1
  Gain5/1 -> Add1/2
  Gain3/1 -> Add1/1
  Gain4/1 -> Vel/1  "GM_2"
  Pos/1 -> Difference/1
  Add1/1 -> Gain4/1, Unit Delay/1

== system QET_KV/Stability Check and Control/Initial and Final Condition Control ==
  Clock : Inport
  is_stable : Inport  Port=2
  Constant1 : Constant  Value=Pos_Init
  Constant2 : Constant  Value=Times
  Constant3 : Constant  Value=Pos_Final
  Constant4 : Constant  Value=100
  Deg to Rad : Gain  Gain=pi/180
  Display : Display
  Enc Interrupt : Scope  NumInputPorts=2
  HIL Poll Interrupt : quarc_library/Data Acquisition/Generic/Interrupts/HIL Poll Interrupt  object_name=HIL-1  channels=[1002]  sample_time=qc_get_step_size  active=on  vector_output=off  data_type_mode=Inherit via back propagation  data_type=boolean
      settings: AttributesFormatString=(%<object_name>)
  MATLAB Function : MATLAB Function  TreatAsAtomicUnit=on
  MATLAB Function1 : MATLAB Function  TreatAsAtomicUnit=on
  Manual Switch : ManualSwitch  CurrentSetting=0
  PD Controller : Subsystem
  Position and Torque : Scope  Commented=on  NumInputPorts=2
  Rad to Deg : Gain  Gain=180/pi
  Rad to Deg1 : Gain  Gain=180/pi
  Transfer Fcn : TransferFcn  Denominator=[1/(2*pi*1) 1]
  Transport Delay : TransportDelay  DelayTime=0.015  InitialOutput=1
  Unit Delay : UnitDelay  SampleTime=-1
  Switch-State : Outport
  Stable Torque : Outport  Port=2
  Pos_PD : Outport  Port=3
  Pos_Final : Outport  Port=4
  tag scope: SwitchSequence=global
  wires:
  [QET2_Pos] -> MATLAB Function1/1(QET_Pos), PD Controller/2(Position), MATLAB Function/4(Pos_in)
  Transfer Fcn/1 -> Pos_PD/1, Position and Torque/1, PD Controller/1(Desired Pos)
  PD Controller/1(Torque) -> Position and Torque/2, Stable Torque/1
  Clock/1 -> MATLAB Function/1(Clock)
  MATLAB Function/3(Pos_out) -> Transfer Fcn/1
  MATLAB Function/1(sw) -> Switch-State/1
  Constant1/1 -> MATLAB Function/3(Pos_Init)
  is_stable/1 -> MATLAB Function/5(is_stable)
  Constant2/1 -> MATLAB Function/2(Times)
  MATLAB Function/2(sw_Sequence) -> Transport Delay/1
  Transport Delay/1 -> [SwitchSequence]
  Manual Switch/1 -> Unit Delay/1, Rad to Deg/1, MATLAB Function/6(Pos_Final)
  Rad to Deg/1 -> Display/1
  Unit Delay/1 -> Pos_Final/1
  Constant3/1 -> MATLAB Function1/2(Pos_Final), Manual Switch/1
  HIL Poll Interrupt/1 -> Enc Interrupt/2, MATLAB Function1/4(INT_Enc)
  Constant4/1 -> Deg to Rad/1
  MATLAB Function1/1(Pos_Final_out) -> Rad to Deg1/1, Manual Switch/2
  Deg to Rad/1 -> MATLAB Function1/3(DesiredPos)
  Rad to Deg1/1 -> Enc Interrupt/1

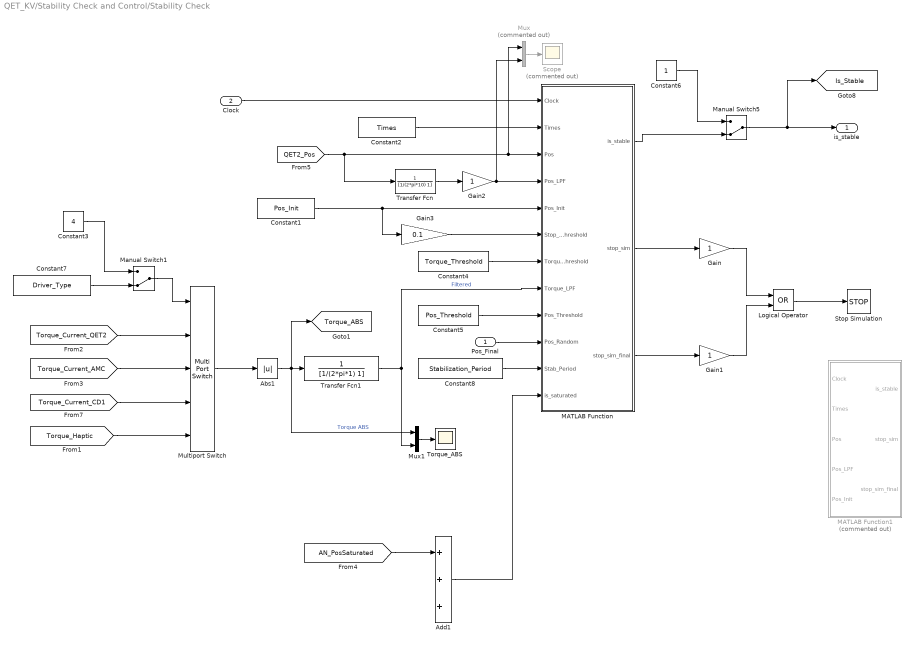
== system QET_KV/Stability Check and Control/Stability Check ==
  Pos_Final : Inport
  Clock : Inport  Port=2
  Abs1 : Abs
  Add1 : Sum  Inputs=+++
  Constant1 : Constant  Value=Pos_Init
  Constant2 : Constant  Value=Times
  Constant3 : Constant  Value=4
  Constant4 : Constant  Value=Torque_Threshold
  Constant5 : Constant  Value=Pos_Threshold
  Constant6 : Constant
  Constant7 : Constant  Value=Driver_Type
  Constant8 : Constant  Value=Stabilization_Period
  Gain : Gain
  Gain1 : Gain
  Gain2 : Gain  SampleTime=qc_get_step_size
  Gain3 : Gain  Gain=0.1  SampleTime=qc_get_step_size
  Logical Operator : Logic  Operator=OR  AllPortsSameDT=off  OutDataTypeStr=boolean
  MATLAB Function : MATLAB Function  TreatAsAtomicUnit=on
  MATLAB Function1 : MATLAB Function  Commented=on  TreatAsAtomicUnit=on
  Manual Switch1 : ManualSwitch  CurrentSetting=0
  Manual Switch5 : ManualSwitch  CurrentSetting=0
  Multiport Switch : MultiPortSwitch  DataPortForDefault=Additional data port  SampleTime=qc_get_step_size
  Mux : Mux  Commented=on  Inputs=2
  Mux1 : Mux  Inputs=2
  Scope : Scope  Commented=on
  Stop Simulation : Stop
  Torque_ABS : Scope
  Transfer Fcn : TransferFcn  Denominator=[1/(2*pi*10) 1]
  Transfer Fcn1 : TransferFcn  Denominator=[1/(2*pi*1) 1]
  is_stable : Outport
  tag scope: Is_Stable=global, Torque_ABS=global
  wires:
  Clock/1 -> MATLAB Function/1(Clock)
  Constant1/1 -> Gain3/1, MATLAB Function/5(Pos_Init)
  MATLAB Function/2(stop_sim) -> Gain/1
  [QET2_Pos] -> Transfer Fcn/1, Mux/1, MATLAB Function/3(Pos)
  Transfer Fcn/1 -> Gain2/1
  Constant2/1 -> MATLAB Function/2(Times)
  Manual Switch5/1 -> is_stable/1, [Is_Stable]
  Gain2/1 -> Mux/2, MATLAB Function/4(Pos_LPF)
  Mux/1 -> Scope/1
  MATLAB Function/1(is_stable) -> Manual Switch5/2
  Constant6/1 -> Manual Switch5/1
  Gain/1 -> Logical Operator/1
  MATLAB Function/3(stop_sim_final) -> Gain1/1
  Gain1/1 -> Logical Operator/2
  Logical Operator/1 -> Stop Simulation/1
  [Torque_Haptic] -> Multiport Switch/5
  [Torque_Current_QET2] -> Multiport Switch/2
  [Torque_Current_AMC] -> Multiport Switch/3
  [Torque_Current_CD1] -> Multiport Switch/4
  Constant7/1 -> Manual Switch1/2
  Constant3/1 -> Manual Switch1/1
  Manual Switch1/1 -> Multiport Switch/1
  Multiport Switch/1 -> Abs1/1
  Mux1/1 -> Torque_ABS/1
  Transfer Fcn1/1 -> Mux1/2, MATLAB Function/8(Torque_LPF)  "Filtered"
  Abs1/1 -> [Torque_ABS], Mux1/1, Transfer Fcn1/1  "Torque ABS"
  Constant4/1 -> MATLAB Function/7(Torque_Threshold)
  Gain3/1 -> MATLAB Function/6(Stop_PosThreshold)
  Constant5/1 -> MATLAB Function/9(Pos_Threshold)
  Pos_Final/1 -> MATLAB Function/10(Pos_Random)
  Constant8/1 -> MATLAB Function/11(Stab_Period)
  Add1/1 -> MATLAB Function/12(is_saturated)
  [AN_PosSaturated] -> Add1/1

== system QET_KV/Stepper Motor/Remove Bias1 ==
  In1 : Inport
  Step : Step  Time=0.5  Before=1  After=0
  Sum1 : Sum  Inputs=|+-
  Switch : Switch  Criteria=u2 > Threshold  Threshold=0.5
  Unit Delay : UnitDelay  SampleTime=-1
  Out1 : Outport
  wires:
  In1/1 -> Switch/1, Sum1/1
  Switch/1 -> Unit Delay/1, Sum1/2
  Step/1 -> Switch/2
  Unit Delay/1 -> Switch/3
  Sum1/1 -> Out1/1

== system QET_KV/Stepper Motor/Stepper Motor Control Absolute ==
  Angle Desired [Deg] : Inport
  PWM Pulses Counter : Inport  Port=2
  Pos Encoder [Deg] : Inport  Port=3
  Clock : Clock
  Constant : Constant  Value=Resolution
  Constant1 : Constant
  Constant7 : Constant
  Display : Display
  Kp : Constant  Value=0.15
  MATLAB Function : MATLAB Function  TreatAsAtomicUnit=on
  MATLAB Function1 : MATLAB Function  Commented=on  TreatAsAtomicUnit=on
  Manual Switch : ManualSwitch
  PWM/DIR : Scope  NumInputPorts=4
  PWM : Outport
  DIR : Outport  Port=2
  ENA : Outport  Port=3
  Pos : Outport  Port=4
  wires:
  Angle Desired [Deg]/1 -> MATLAB Function/1(Pos_Ref)
  Constant/1 -> MATLAB Function/5(Resolution)
  MATLAB Function/4(Pos_out) -> Pos/1
  PWM Pulses Counter/1 -> MATLAB Function/2(Pos_Counter)
  MATLAB Function/5(e) -> PWM/DIR/3
  Kp/1 -> MATLAB Function/6(Kp)
  MATLAB Function/1(PWM) -> PWM/1, PWM/DIR/1
  MATLAB Function/2(DIR) -> PWM/DIR/2, DIR/1
  Pos Encoder [Deg]/1 -> MATLAB Function/3(Pos_Enc_Deg)
  Constant7/1 -> MATLAB Function/4(Pos_Select)
  Constant1/1 -> Manual Switch/2
  Manual Switch/1 -> MATLAB Function/7(Clock)
  Clock/1 -> Manual Switch/1, Display/1
  MATLAB Function/6(Res_Bias) -> PWM/DIR/4
  MATLAB Function/3(ENA) -> ENA/1

== system QET_KV/Virtual Environment/VE_KV_BD ==
  Position : Inport
  Add : Sum  Inputs=--
  Discrete Derivative : simulink/Discrete/Discrete Derivative  gainval=1.0  ICPrevScaledInput=0.0  InputProcessing=Inherited  OutMin=[]  OutMax=[]  OutDataType=fixdt(1, 16)  OutScaling=2^-10  DoSatur=off
  Gain : Gain  Gain=K
  Gain1 : Gain  Gain=B - Kappa
  Torque : Outport
  tag scope: QET_Vel_BD=global
  wires:
  Gain1/1 -> Add/2
  Discrete Derivative/1 -> [QET_Vel_BD], Gain1/1
  Gain/1 -> Add/1
  Add/1 -> Torque/1
  Position/1 -> Discrete Derivative/1, Gain/1

== system QET_KV/Virtual Environment/VE_KV_GM2 ==
  Position : Inport
  Add : Sum  Inputs=--  SampleTime=Ts_loop
  Discrete Transfer Fcn : DiscreteTransferFcn  Numerator=[1 -1]  Denominator=[Delta Delta*lambda]  SampleTime=Ts_loop
  Discrete Derivative : simulink/Discrete/Discrete Derivative  gainval=1.0  ICPrevScaledInput=0.0  InputProcessing=Inherited  OutMin=[]  OutMax=[]  OutDataType=fixdt(1, 16)  OutScaling=2^-10  DoSatur=off
  GM : Subsystem
  Gain : Gain  Gain=K  SampleTime=Ts_loop
  Gain1 : Gain  Gain=B - Kappa  SampleTime=Ts_loop
  Gain2 : Gain  Gain=1/mag  SampleTime=Ts_loop
  Manual Switch4 : ManualSwitch  CurrentSetting=0  SampleTime=Ts_loop
  Mux2 : Mux  Inputs=3
  Rate Transition : RateTransition  Integrity=off  Deterministic=off  OutPortSampleTime=Ts_loop
  Rate Transition1 : RateTransition  Integrity=off  Deterministic=off  OutPortSampleTime=Ts
  Rate Transition2 : RateTransition  Integrity=off  Deterministic=off  OutPortSampleTime=Ts
  Velocities : Scope
  Torque : Outport
  tag scope: QET_Vel_GM=global
  wires:
  Gain1/1 -> Add/2
  Discrete Transfer Fcn/1 -> Gain2/1
  Gain/1 -> Add/1
  Add/1 -> Rate Transition1/1
  Position/1 -> Rate Transition/1
  Mux2/1 -> Velocities/1
  GM/1(Vel) -> Manual Switch4/2, Mux2/2  "GM_2"
  Discrete Derivative/1 -> Mux2/3  "BD"
  Gain2/1 -> Mux2/1, Manual Switch4/1  "GM"
  Rate Transition/1 -> Gain/1, Discrete Transfer Fcn/1, GM/1(Pos), Discrete Derivative/1
  Rate Transition1/1 -> Torque/1
  Rate Transition2/1 -> [QET_Vel_GM]
  Manual Switch4/1 -> Gain1/1, Rate Transition2/1

== system QET_KV/Virtual Environment/VE_PV ==
  Position : Inport
  Velocity : Inport  Port=2
  Add : Sum  Inputs=--  SampleTime=Ts_loop
  Gain : Gain  Gain=K  SampleTime=Ts_loop
  Gain1 : Gain  Gain=B - Kappa  SampleTime=Ts_loop
  Rate Transition : RateTransition  Integrity=off  Deterministic=off  OutPortSampleTime=Ts_loop
  Rate Transition1 : RateTransition  Integrity=off  Deterministic=off  OutPortSampleTime=Ts
  Rate Transition2 : RateTransition  Integrity=off  Deterministic=off  OutPortSampleTime=Ts_loop
  Torque : Outport
  wires:
  Gain1/1 -> Add/2
  Gain/1 -> Add/1
  Add/1 -> Rate Transition1/1
  Position/1 -> Rate Transition/1
  Rate Transition2/1 -> Gain1/1
  Rate Transition/1 -> Gain/1
  Rate Transition1/1 -> Torque/1
  Velocity/1 -> Rate Transition2/1

== system QET_KV/Analog VE/Digital Outputs/Clock Pulses ==
  Time [s] : Inport
  Width [s] : Inport  Port=2
  Add : Sum
  Clock : Clock
  Logical Operator : Logic  Operator=NOT  AllPortsSameDT=off  OutDataTypeStr=boolean
  Memory : Memory
  Product : Product  Inputs=3  SampleTime=Ts
  Relational Operator : RelationalOperator  OutDataTypeStr=boolean
  Relational Operator1 : RelationalOperator  Operator=<=  OutDataTypeStr=boolean
  Out1 : Outport
  wires:
  Clock/1 -> Relational Operator1/1, Relational Operator/1
  Time [s]/1 -> Add/1, Relational Operator/2
  Width [s]/1 -> Add/2
  Add/1 -> Relational Operator1/2
  Relational Operator/1 -> Product/2
  Relational Operator1/1 -> Product/3
  Product/1 -> Out1/1
  Memory/1 -> Logical Operator/1
  Logical Operator/1 -> Product/1, Memory/1

== system QET_KV/Analog VE/Digital Outputs/Pulse ==
  Amplitude : Inport
  Time [s] : Inport  Port=2
  Width [s] : Inport  Port=3
  Add : Sum
  Clock : Clock
  Product : Product  Inputs=3
  Relational Operator : RelationalOperator  OutDataTypeStr=boolean
  Relational Operator1 : RelationalOperator  Operator=<=  OutDataTypeStr=boolean
  Out1 : Outport
  wires:
  Clock/1 -> Relational Operator1/1, Relational Operator/1
  Time [s]/1 -> Add/1, Relational Operator/2
  Width [s]/1 -> Add/2
  Add/1 -> Relational Operator1/2
  Relational Operator/1 -> Product/2
  Relational Operator1/1 -> Product/3
  Product/1 -> Out1/1
  Amplitude/1 -> Product/1

== system QET_KV/Analog VE/Digital Outputs/Time Enable2 ==
  In1 : Inport
  Product2 : Product  Inputs=3
  Step4 : Step  Time=0.1  SampleTime=Ts
  Step5 : Step  Time=Chirp_Period+1.5  Before=1  After=0  SampleTime=Ts
  Out1 : Outport
  wires:
  Step5/1 -> Product2/3
  Product2/1 -> Out1/1
  In1/1 -> Product2/1
  Step4/1 -> Product2/2

== system QET_KV/Analog VE/Digital Outputs/Unit Pulse ==
  Time [s] : Inport
  Width [s] : Inport  Port=2
  Add : Sum
  Clock : Clock
  Constant : Constant
  Product : Product  Inputs=3
  Relational Operator : RelationalOperator  OutDataTypeStr=boolean
  Relational Operator1 : RelationalOperator  Operator=<=  OutDataTypeStr=boolean
  Out1 : Outport
  wires:
  Clock/1 -> Relational Operator1/1, Relational Operator/1
  Time [s]/1 -> Add/1, Relational Operator/2
  Width [s]/1 -> Add/2
  Add/1 -> Relational Operator1/2
  Relational Operator/1 -> Product/2
  Relational Operator1/1 -> Product/3
  Product/1 -> Out1/1
  Constant/1 -> Product/1

== system QET_KV/Analog VE/Digital Outputs/Unit Pulse1 ==
  Time [s] : Inport
  Width [s] : Inport  Port=2
  Add : Sum
  Clock : Clock
  Constant1 : Constant
  Product : Product  Inputs=3
  Relational Operator : RelationalOperator  OutDataTypeStr=boolean
  Relational Operator1 : RelationalOperator  Operator=<=  OutDataTypeStr=boolean
  Out1 : Outport
  wires:
  Clock/1 -> Relational Operator1/1, Relational Operator/1
  Time [s]/1 -> Add/1, Relational Operator/2
  Width [s]/1 -> Add/2
  Add/1 -> Relational Operator1/2
  Relational Operator/1 -> Product/2
  Relational Operator1/1 -> Product/3
  Product/1 -> Out1/1
  Constant1/1 -> Product/1

== system QET_KV/Analog VE/GBC Method/S//H Block ==
  Input : Inport
  S/H : Inport  Port=2
  Multiport Switch : MultiPortSwitch  DataPortOrder=Specify indices  Inputs=2  DataPortIndices={0,1}  SampleTime=qc_get_step_size
  Unit Delay : UnitDelay  SampleTime=qc_get_step_size
  Output : Outport
  wires:
  Input/1 -> Multiport Switch/3
  S/H/1 -> Multiport Switch/1
  Multiport Switch/1 -> Unit Delay/1, Output/1
  Unit Delay/1 -> Multiport Switch/2

== system QET_KV/Analog VE/GBC Method -WHC/S//H Block ==
  Input : Inport
  S/H : Inport  Port=2
  Multiport Switch : MultiPortSwitch  DataPortOrder=Specify indices  Inputs=2  DataPortIndices={0,1}  SampleTime=qc_get_step_size
  Unit Delay : UnitDelay  SampleTime=qc_get_step_size
  Output : Outport
  wires:
  Input/1 -> Multiport Switch/3
  S/H/1 -> Multiport Switch/1
  Multiport Switch/1 -> Unit Delay/1, Output/1
  Unit Delay/1 -> Multiport Switch/2

== system QET_KV/Haptic_System/Driver Voltage or Current/Motor equation ==
  Torque : Inport
  Vel : Inport  Port=2
  Divide : Product  Inputs=*/  SampleTime=Ts
  Ka : Constant  Value=0.0502  SampleTime=Ts
  Kemf : Gain  Gain=0.0502  SampleTime=Ts
  R : Gain  Gain=10.6  SampleTime=Ts
  Scope : Scope  Commented=on  NumInputPorts=2
  Sum : Sum  Inputs=|++
  Voltage : Outport
  wires:
  Ka/1 -> Divide/2
  R/1 -> Divide/1
  Kemf/1 -> Scope/2, Sum/2
  Torque/1 -> R/1
  Vel/1 -> Kemf/1
  Sum/1 -> Voltage/1
  Divide/1 -> Scope/1, Sum/1

== system QET_KV/Stability Check and Control/Initial and Final Condition Control/PD Controller ==
  Desired Pos : Inport
  Position : Inport  Port=2
  Discrete Derivative : simulink/Discrete/Discrete Derivative  gainval=1.0  ICPrevScaledInput=0.0  InputProcessing=Inherited  OutMin=[]  OutMax=[]  OutDataType=fixdt(1, 16)  OutScaling=2^-10  DoSatur=off
  Discrete Derivative1 : simulink/Discrete/Discrete Derivative  gainval=1.0  ICPrevScaledInput=0.0  InputProcessing=Inherited  OutMin=[]  OutMax=[]  OutDataType=fixdt(1, 16)  OutScaling=2^-10  DoSatur=off
  Gain : Gain  Gain=Kp
  Gain1 : Gain  Gain=Kd
  Kp Kd Torque : Scope  Commented=on  NumInputPorts=2
  Manual Switch5 : ManualSwitch  CurrentSetting=0
  Mux1 : Mux  Commented=on  Inputs=2
  Rate Transition : RateTransition  Integrity=off  OutPortSampleTime=Ts*2
  Rate Transition1 : RateTransition  Integrity=off  OutPortSampleTime=Ts
  Sum : Sum  Inputs=|+-
  Sum1 : Sum  Inputs=|+-
  Transfer Fcn : TransferFcn  Denominator=[1/(2*pi*1) 1]
  Torque : Outport
  Velocity [rad/s] : Outport  Port=2
  wires:
  Position/1 -> Sum/2, Discrete Derivative1/1, Rate Transition/1
  Desired Pos/1 -> Sum/1
  Sum/1 -> Gain/1
  Discrete Derivative/1 -> Rate Transition1/1
  Sum1/1 -> Kp Kd Torque/2, Torque/1
  Mux1/1 -> Kp Kd Torque/1
  Gain/1 -> Sum1/1, Mux1/1
  Gain1/1 -> Mux1/2, Sum1/2
  Rate Transition/1 -> Discrete Derivative/1
  Transfer Fcn/1 -> Manual Switch5/1
  Rate Transition1/1 -> Transfer Fcn/1
  Manual Switch5/1 -> Velocity [rad/s]/1, Gain1/1
  Discrete Derivative1/1 -> Manual Switch5/2

== system QET_KV/Virtual Environment/VE_KV_GM2/GM ==
  Pos : Inport
  Add1 : Sum  Inputs=+-  SampleTime=Ts_loop
  Difference : simulink/Discrete/Difference  ICPrevInput=0.0  InputProcessing=Inherited  OutMin=[]  OutMax=[]  OutDataType=fixdt(1, 16)  OutScaling=2^-10  DoSatur=off
  Gain3 : Gain  Gain=1/Delta  SampleTime=Ts_loop
  Gain4 : Gain  Gain=1/mag  SampleTime=Ts_loop
  Gain5 : Gain  Gain=lambda  SampleTime=Ts_loop
  Unit Delay : UnitDelay  SampleTime=Ts_loop
  Vel : Outport
  wires:
  Unit Delay/1 -> Gain5/1
  Difference/1 -> Gain3/1
  Gain5/1 -> Add1/2
  Gain3/1 -> Add1/1
  Gain4/1 -> Vel/1  "GM_2"
  Pos/1 -> Difference/1
  Add1/1 -> Gain4/1, Unit Delay/1

== matlab function QET_KV/PSoC Comm/MATLAB Function ==
  data: K input; B input; Freq input; X input; M input; C input; cmd output uint8; en output
function [cmd, en] = fcn(K,B,Freq,X,M,C)
%#codegen

persistent K_last B_last X_last C_last Freq_last M_last
if (isempty(K_last))
    K_last = K; B_last = B;
    X_last = 0; C_last = 5;
    Freq_last = 0;
    M_last = 0;
end
%cmd = cast('     ','uint8');
sum_ = 0;
cmd = uint8(zeros(1,6));
en = 0;
%%
if (abs(K - K_last) > 1e-8)
    K_last = K;
    cmd(1) = uint8('K');
    cmd(2:5) = typecast(single(K),'uint8');
    en = 1;
    
elseif (abs(B - B_last) > 1e-8)
    B_last = B;
    cmd(1) = uint8('B');
    cmd(2:5) = typecast(single(B),'uint8');
    en = 1;
    
elseif (abs(Freq - Freq_last) > 1e-8)
    Freq_last = Freq;
    cmd(1) = uint8('F');
    cmd(2:5) = typecast(single(Freq),'uint8');
    en = 1;
    
elseif (abs(X - X_last) > 1e-8)
    X_last = X;
    cmd(1) = uint8('X');
    cmd(2:5) = typecast(single(X),'uint8');
    en = 1;
    
elseif (abs(M - M_last) > 1e-3)
    M_last = M;
    cmd(1) = uint8('M');
    cmd(2) = uint8(M);
    en = 1;
    
elseif (abs(C - C_last) > 1e-3)
    C_last = C;
    
    cmd(1) = uint8('C');
    cmd(2) = uint8(C);
    en = 1;
end
%%
if (en == 1)
    sum_ = mod(sum(cmd),256);
    cmd(6) = 255-sum_;
end
